simulink library "powerlib2"  (Simulink 6.0)
settings: Solver=ode45  SolverMode=SingleTasking  StartTime=0.0  StopTime=10.0  RelTol=1e-3
undefined symbols (not defined in the file or in its folder): com, ctrl1, Da, DiscIntNeverNeededParam, dtha, etat, FA, gcbh, Ha, Ka, Lm, Ls, powericonV2, q0, Rm, Rs, sel, st_a, st_b, st_c, sta, stb, stc, T1, T2, T3, T4
libraries: powerlib2 x55, simulink_extras x5, powerlib_extras x4, powerlib_modelsV2 x4, simulink x1
(part 5 of 6)

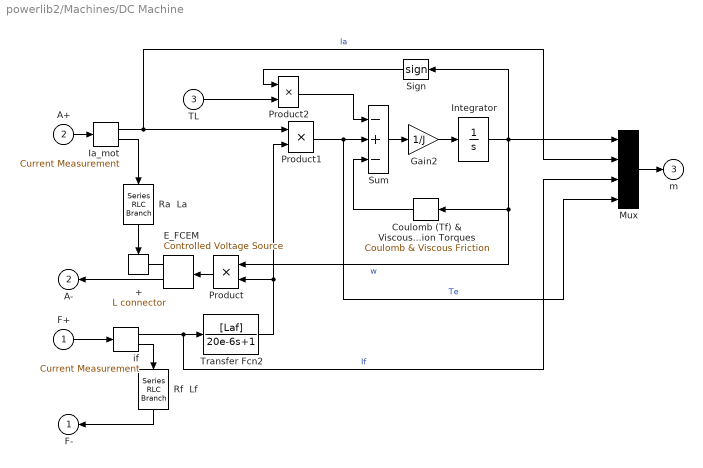
== system powerlib2/Machines/DC Machine ==
  F+ : Inport  Port=1  LatchInput=off
  A+ : Inport  Port=2  LatchInput=off
  TL : Inport  Port=3  LatchInput=off
  + : powerlib2/Connectors/L connector  Tag=PoWeRsYsTeMbLoCk  Orientation=down
  Coulomb (Tf) & Viscous ( Bm*w)  Friction Torques : simulink/Discontinuities/Coulomb & Viscous Friction  Orientation=left  offset=Tf  gain=Bm
  E_FCEM : powerlib2/Electrical Sources/Controlled Voltage Source  Tag=PoWeRsYsTeMbLoCk  Orientation=left  initsrc=on  srctyp=AC  iv=0  iph=0  ifreq=0  mesure=None  PSBOutputType=11
  Gain2 : Gain  Gain=1/J  SaturateOnIntegerOverflow=on
  Ia_mot : powerlib2/Measurements/Current Measurement  Tag=PoWeRsYsTeMmEaSuReMeNtFiRsT  PhasorSimulation=off  OutputType=Magnitude  PSBOutputType=01  PSBequivalent=0
  Integrator : Integrator  InitialCondition=w0
  Mux : Mux
  Product : Product  Orientation=left  SaturateOnIntegerOverflow=on  InputSameDT=on
  Product1 : Product  SaturateOnIntegerOverflow=on  InputSameDT=on
  Product2 : Product  SaturateOnIntegerOverflow=on  InputSameDT=on
  Ra  La : powerlib2/Elements/Series RLC Branch  Tag=PoWeRsYsTeMbLoCk  Orientation=down  a=Ra  b=La  c=inf  mesure=None  PSBOutputType=1
  Rf  Lf : powerlib2/Elements/Series RLC Branch  Tag=PoWeRsYsTeMbLoCk  Orientation=down  a=Rf  b=Lf  c=inf  mesure=None  PSBOutputType=1
  Sign : Signum  Orientation=left
  Sum : Sum  Inputs=-+-  SaturateOnIntegerOverflow=on  InputSameDT=on
  Transfer Fcn2 : TransferFcn  Numerator=[Laf]  Denominator=[20e-6 1]
  if : powerlib2/Measurements/Current Measurement  Tag=PoWeRsYsTeMmEaSuReMeNt  PhasorSimulation=off  OutputType=Magnitude  PSBOutputType=01  PSBequivalent=0
  F- : Outport  Orientation=left  InitialOutput=0
  A- : Outport  Orientation=left  Port=2  InitialOutput=0
  m : Outport  Port=3  InitialOutput=0
  wires:
  A+/1 -> Ia_mot/1
  Ia_mot/2 -> Ra  La/1
  Ra  La/1 -> +/1
  F+/1 -> if/1
  if/2 -> Rf  Lf/1
  E_FCEM/1 -> +/Enable
  E_FCEM/2 -> A-/1
  Rf  Lf/1 -> F-/1
  Ia_mot/1 -> Product1/1, Mux/2  "Ia"
  if/1 -> Transfer Fcn2/1, Mux/3  "If"
  Product2/1 -> Sum/1
  TL/1 -> Product2/2
  Sign/1 -> Product2/1
  Sum/1 -> Gain2/1
  Gain2/1 -> Integrator/1
  Integrator/1 -> Coulomb (Tf) & Viscous ( Bm*w)  Friction Torques/1, Product/1, Mux/1, Sign/1  "w"
  Product/1 -> E_FCEM/1
  Product1/1 -> Sum/2, Mux/4  "Te"
  Mux/1 -> m/1
  Transfer Fcn2/1 -> Product1/2, Product/2
  Coulomb (Tf) & Viscous ( Bm*w)  Friction Torques/1 -> Sum/3

== system powerlib2/Machines/Excitation System ==
  vref : Inport  Port=1  LatchInput=off
  vd : Inport  Port=2  LatchInput=off
  vq : Inport  Port=3  LatchInput=off
  vstab : Inport  Port=4  LatchInput=off
  Source : powerlib_modelsV2/Continuous/Excitation_System  tr=tr  reg=reg  exc=exc  tgr=tgr  damp=damp  sat=sat  lim=lim  v0=v0
  Vf : Outport  InitialOutput=0
  wires:
  Source/1 -> Vf/1
  vref/1 -> Source/1
  vd/1 -> Source/2
  vq/1 -> Source/3
  vstab/1 -> Source/4

== system powerlib2/Machines/Generic Power System Stabilizer ==
  In : Inport  Port=1  LatchInput=off
  Source : powerlib_modelsV2/Continuous/PSS  Tsensor=Tsensor  K=K  Twashout=Twashout  Tleadlag1=Tleadlag1  Tleadlag2=Tleadlag2  VSlimits=VSlimits  Vinit=Vinit  Plot_On=off  MagdB_On=on  FreqRange=logspace(-2,2,500)
  Vstab : Outport  InitialOutput=0
  wires:
  Source/1 -> Vstab/1
  In/1 -> Source/1

== system powerlib2/Machines/HTG ==
  wref : Inport  Port=1  LatchInput=off
  Pref : Inport  Port=2  LatchInput=off
  we : Inport  Port=3  LatchInput=off
  Pe0 : Inport  Port=4  LatchInput=off
  dw : Inport  Port=5  LatchInput=off
  Source : powerlib_modelsV2/Continuous/HTG  sm=sm  gate=gate  reg=reg  hyd=hyd  dref=dref  po=po
  Pm : Outport  InitialOutput=0
  gate : Outport  Port=2  InitialOutput=0
  wires:
  wref/1 -> Source/1
  Pref/1 -> Source/2
  we/1 -> Source/3
  Pe0/1 -> Source/4
  dw/1 -> Source/5
  Source/2 -> gate/1
  Source/1 -> Pm/1

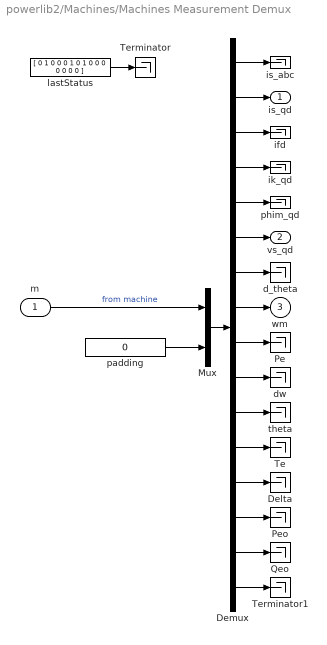
== system powerlib2/Machines/Machines Measurement Demux ==
  m : Inport  Port=1  LatchInput=off
  Delta : Terminator
      settings: Tag=port13
  Demux : Demux  Outputs="[3 2 1 3 2 2 1 1 1 1 1 1 1 1 1,  1]"
  Mux : Mux  Inputs=2
  Pe : Terminator
      settings: Tag=port9
  Peo : Terminator
      settings: Tag=port14
  Qeo : Terminator
      settings: Tag=port15
  Te : Terminator
      settings: Tag=port12
  Terminator : Terminator
  Terminator1 : Terminator
  d_theta : Terminator
      settings: Tag=port7
  dw : Terminator
      settings: Tag=port10
  ifd : Terminator
      settings: Tag=port3
  ik_qd : Terminator
      settings: Tag=port4
  is_abc : Terminator
      settings: Tag=port1
  lastStatus : Constant  Value="[ 0  1  0  0  0  1  0  1  0  0  0  0  0  0  0 ]"
  padding : Constant  Value=0
  phim_qd : Terminator
      settings: Tag=port5
  theta : Terminator
      settings: Tag=port11
  is_qd : Outport  Tag=port2
  vs_qd : Outport  Tag=port6  Port=2
  wm : Outport  Tag=port8  Port=3
  wires:
  padding/1 -> Mux/2
  Demux/1 -> is_abc/1
  Demux/2 -> is_qd/1
  Demux/3 -> ifd/1
  Demux/4 -> ik_qd/1
  Demux/5 -> phim_qd/1
  Demux/6 -> vs_qd/1
  Demux/7 -> d_theta/1
  Demux/8 -> wm/1
  Demux/9 -> Pe/1
  Demux/10 -> dw/1
  Demux/11 -> theta/1
  Mux/1 -> Demux/1
  lastStatus/1 -> Terminator/1
  m/1 -> Mux/1  "from machine"
  Demux/16 -> Terminator1/1
  Demux/15 -> Qeo/1
  Demux/14 -> Peo/1
  Demux/13 -> Delta/1
  Demux/12 -> Te/1

== system powerlib2/Machines/Multi-Band Power System Stabilizer ==
  dw : Inport  Port=1  LatchInput=off
  Source : powerlib_modelsV2/Continuous/MBPSS  OperationMode=Simplified settings  Kg=Kg  GL=GL  GI=GI  GH=GH  GLd=GLd  TcLF=TcLF  GId=GId  TcIF=TcIF  GHd=GHd  TcHF=TcHF  LIM=LIM  Plot_On=off  MagdB_On=off  FreqRange=logspace(-2,2,500)
  Vstab : Outport  InitialOutput=0
  wires:
  dw/1 -> Source/1
  Source/1 -> Vstab/1

== system powerlib2/Machines/Permanent Magnet Synchronous Machine ==
  A : Inport  Port=1  LatchInput=off
  B : Inport  Port=2  LatchInput=off
  C : Inport  Port=3  LatchInput=off
  Tm : Inport  Port=4  LatchInput=off
  Terminator : Terminator
  Terminator1 : Terminator
  Terminator2 : Terminator
  m : Outport  InitialOutput=0
  tag scope: tp200482=global
  wires:
  C/1 -> Terminator2/1
  B/1 -> Terminator1/1
  A/1 -> Terminator/1
  Tm/1 -> [tp200482]
  [tp200488] -> m/1

== system powerlib2/Machines/STG ==
  wref : Inport  Port=1  LatchInput=off
  Pref : Inport  Port=2  LatchInput=off
  wm : Inport  Port=3  LatchInput=off
  d_theta : Inport  Port=4  LatchInput=off
  4 mass shaft : Subsystem  TreatAsAtomicUnit=on
  Constant2 : Constant  Orientation=up  Value=gentype==2
  Constant3 : Constant  Orientation=up  Value=gentype~=2
  Pboil : Constant  Orientation=left  Value=1.0
  Product : Product  SaturateOnIntegerOverflow=on  InputSameDT=on
  Sum : Sum  Inputs=+  SaturateOnIntegerOverflow=on  InputSameDT=on
  Switch1 : Switch  Threshold=0.5  InputSameDT=on
  speed regulator : Subsystem  mask(Speed regulator for thermal turbine){Rp=reg1(2), Kp=reg1(1), Dz=reg1(3), Tsr=reg2(1), Tsm=reg2(2), lim=reg3, g0=q0}
      mask prompts: Rp "Permanent droop Rp:"; Kp "Regulator gain Kp:"; Dz "Regulator dead zone limit Dz (p.u.):"; Tsr "Speed relay time constant Tsr (s):"; Tsm "Servo motor time constant Tsv:"; lim "Gate opening limits [ vgmin,vgmax (p.u./s)  gmin,gmax (p.u.)]:"; g0 "Initial gate opening g0 (p.u.):"
      mask init:
      | vgmin=lim(1); vgmax=lim(2); gmin=lim(3); gmax=lim(4);
  steam turbine : Subsystem  mask(Thermal turbine){Fa=FA, Ta=turb1, f0=q0}
      mask prompts: Fa "Generator 1 torque fractions [ F1  F2  F3  F4 ]:"; Ta "Time constants [ T1  T2  T3  T4 ] (s):"; f0 "Initial flows f0:"
      mask init:
      | F2=Fa(1); F3=Fa(2); F4=Fa(3); F5=Fa(4);
      | if Ta(1)==0, T1=1; else T1=Ta(1); end; if Ta(2)==0, T2=1; else T2=Ta(2); end
      | if Ta(3)==0, T3=1; else T3=Ta(3); end; if Ta(4)==0, T4=1; else T4=Ta(4); end
  dw_5-2 : Outport
  Tr5-2 : Outport  Port=2
  gate : Outport  Port=3
  Pm : Outport  Port=4
  wires:
  wm/1 -> Product/2, speed regulator/4(w)
  Pref/1 -> speed regulator/2(Pref)
  wref/1 -> speed regulator/3(wref)
  Pboil/1 -> steam turbine/2(Pboil)
  Product/1 -> Pm/1
  4 mass shaft/2(Tr2-5) -> Tr5-2/1
  Switch1/1 -> Product/1
  4 mass shaft/1(Tm_g) -> Switch1/3
  Sum/1 -> Switch1/1
  Constant3/1 -> Switch1/2
  d_theta/1 -> 4 mass shaft/2(d_theta)
  steam turbine/1(flowHp) -> speed regulator/1(flowHP)
  steam turbine/2(T5-2) -> 4 mass shaft/1(T5-2), Sum/1
  4 mass shaft/3(dw_5-2) -> dw_5-2/1
  speed regulator/1(gate opening) -> steam turbine/1(gate), gate/1
  Constant2/1 -> 4 mass shaft/Enable

== system powerlib2/Machines/Simplified Synchronous  Machine  pu Units ==
  Pm : Inport  Port=1  LatchInput=off
  E : Inport  Port=2  LatchInput=off
  Constant{,1..3} (4 alike) : Constant
  N : Terminator
  A : Outport  InitialOutput=0
  B : Outport  Port=2  InitialOutput=0
  C : Outport  Port=3  InitialOutput=0
  m_pu : Outport  Port=4  InitialOutput=0
  tag scope: tp200493=global, tp200499=global
  wires:
  [tp200504] -> m_pu/1
  Constant3/1 -> N/1
  Pm/1 -> [tp200493]
  E/1 -> [tp200499]
  Constant2/1 -> C/1
  Constant1/1 -> B/1
  Constant/1 -> A/1

== system powerlib2/Machines/Simplified Synchronous  Machine SI Units ==
  Pm : Inport  Port=1  LatchInput=off
  E : Inport  Port=2  LatchInput=off
  Constant{,1..3} (4 alike) : Constant
  N : Terminator
  A : Outport  InitialOutput=0
  B : Outport  Port=2  InitialOutput=0
  C : Outport  Port=3  InitialOutput=0
  m_SI : Outport  Port=4  InitialOutput=0
  tag scope: tp200509=global, tp200515=global
  wires:
  Constant3/1 -> N/1
  Constant2/1 -> C/1
  [tp200521] -> m_SI/1
  Constant/1 -> A/1
  Constant1/1 -> B/1
  Pm/1 -> [tp200509]
  E/1 -> [tp200515]

== system powerlib2/Machines/Synchronous Machine SI Fundamental ==
  Pm : Inport  Port=1  LatchInput=off
  Vf : Inport  Port=2  LatchInput=off
  Constant : Constant
  Constant1 : Constant
  Constant2 : Constant
  A : Outport  InitialOutput=0
  B : Outport  Port=2  InitialOutput=0
  C : Outport  Port=3  InitialOutput=0
  m_SI : Outport  Port=4  InitialOutput=0
  tag scope: tp200526=global, tp200532=global
  wires:
  Vf/1 -> [tp200532]
  Pm/1 -> [tp200526]
  [tp200537] -> m_SI/1
  Constant/1 -> A/1
  Constant1/1 -> B/1
  Constant2/1 -> C/1

== system powerlib2/Machines/Synchronous Machine pu Fundamental ==
  Pm : Inport  Port=1  LatchInput=off
  Vf : Inport  Port=2  LatchInput=off
  Constant : Constant
  Constant1 : Constant
  Constant2 : Constant
  A : Outport  InitialOutput=0
  B : Outport  Port=2  InitialOutput=0
  C : Outport  Port=3  InitialOutput=0
  m_pu : Outport  Port=4  InitialOutput=0
  tag scope: tp200543=global, tp200548=global
  wires:
  [tp200554] -> m_pu/1
  Pm/1 -> [tp200543]
  Vf/1 -> [tp200548]
  Constant/1 -> A/1
  Constant1/1 -> B/1
  Constant2/1 -> C/1

== system powerlib2/Machines/Synchronous Machine pu Standard ==
  Pm : Inport  Port=1  LatchInput=off
  Vf : Inport  Port=2  LatchInput=off
  Constant : Constant
  Constant1 : Constant
  Constant2 : Constant
  A : Outport  InitialOutput=0
  B : Outport  Port=2  InitialOutput=0
  C : Outport  Port=3  InitialOutput=0
  m_pu : Outport  Port=4  InitialOutput=0
  tag scope: tp200559=global, tp200565=global
  wires:
  Vf/1 -> [tp200565]
  Pm/1 -> [tp200559]
  [tp200570] -> m_pu/1
  Constant/1 -> A/1
  Constant1/1 -> B/1
  Constant2/1 -> C/1

== system powerlib2/Measurements/Current Measurement ==
  + : Inport  Port=1  LatchInput=off
  Constant : Constant  Orientation=left
  Mux : Mux  Inputs=2
  Phasor Measurements : powerlib2/Measurements/Voltage Measurement/Phasor Measurements  TreatAsAtomicUnit=on  SimViewingDevice=off  DataTypeOverride=UseLocalSettings  MinMaxOverflowLogging=UseLocalSettings
      settings: Permissions=ReadWrite  RTWFcnNameOpts=Auto  RTWFileNameOpts=Auto
  Selector : Selector  Elements=SelectionMode  InputPortWidth=length(OutputSelection)+1
  Simulation method : Constant  Orientation=down  Value=PhasorSimulation
  Terminator : Terminator
  i : Outport  InitialOutput=0
  - : Outport  Orientation=left  Port=2  InitialOutput=0
  wires:
  +/1 -> Terminator/1
  Constant/1 -> -/1
  Simulation method/1 -> Phasor Measurements/Enable
  Mux/1 -> Selector/1
  Phasor Measurements/1 -> Mux/1
  [tp200576] -> Phasor Measurements/1, Mux/2
  Selector/1 -> i/1

== system powerlib2/Measurements/Extra Library  ==

== system powerlib2/Measurements/Extra Library 1 ==

== system powerlib2/Measurements/Impedance Measurement ==
  note: Use this block
      | with the powergui
      | interface
  1 : Inport  Port=1  LatchInput=off
  2 : Inport  Port=2  LatchInput=off
  Terminator : Terminator
  Terminator1 : Terminator
  wires:
  2/1 -> Terminator1/1
  1/1 -> Terminator/1

== system powerlib2/Measurements/Multimeter ==
  Gain2 : Gain  Gain=Gain  SaturateOnIntegerOverflow=on
  Mode : Constant  Value=Display
  Mux : Mux  Inputs=2
  Phasor Measurements : Subsystem  TreatAsAtomicUnit=on
  Selector : Selector  Elements=SelectionMode  InputPortWidth=length(OutputSelection)+length(sel)
  Simulation method : Constant  Orientation=down  Value=PhasorSimulation
  StoreData : Subsystem  Orientation=down  LoadFcn=if strcmp(bdroot,'powerlib')|strcmp(bdroot,'powerlib11')|strcmp(bdroot,'powerlib2');return;else;set_param([gcb,'/To Workspace'],'VariableName',strrep(tempname,tempdir,''));end  TreatAsAtomicUnit=on  mask{RowMax=inf}
      mask prompts: RowMax "Maximum Number of rows"
      settings: CopyFcn=if strcmp(bdroot,'powerlib')|strcmp(bdroot,'powerlib11')|strcmp(bdroot,'powerlib2');return;else;set_param([gcb,'/To Workspace'],'VariableName',strrep(tempname,tempdir,''));end
  selection : Selector  Elements=sel  InputPortWidth=L
  Out1 : Outport
  wires:
  Mode/1 -> StoreData/Enable
  selection/1 -> Gain2/1
  [gotomultimeterPSB] -> selection/1
  Gain2/1 -> Phasor Measurements/1(In1), Mux/2
  Simulation method/1 -> Phasor Measurements/Enable
  Phasor Measurements/1(Out1) -> Mux/1
  Mux/1 -> Selector/1
  Selector/1 -> Out1/1, StoreData/1(In1)

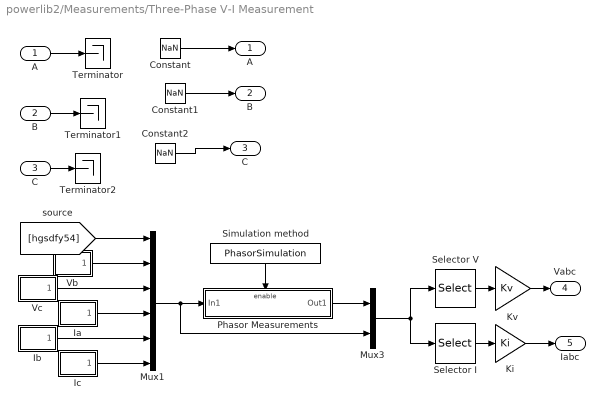
== system powerlib2/Measurements/Three-Phase V-I Measurement ==
  A : Inport  Port=1  LatchInput=off
  B : Inport  Port=2  LatchInput=off
  C : Inport  Port=3  LatchInput=off
  Constant : Constant  Value=NaN
  Constant1 : Constant  Value=NaN
  Constant2 : Constant  Value=NaN
  Ia : Subsystem
  Ib : Subsystem
  Ic : Subsystem
  Ki : Gain  Gain=Ki  SaturateOnIntegerOverflow=on
  Kv : Gain  Gain=Kv  SaturateOnIntegerOverflow=on
  Mux1 : Mux  Inputs=6
  Mux3 : Mux  Inputs=2
  Phasor Measurements : Subsystem  TreatAsAtomicUnit=on
  Selector I : Selector  Elements=SelectionModeI  InputPortWidth=length(OutputSelection)+6
  Selector V : Selector  Elements=SelectionModeV  InputPortWidth=length(OutputSelection)+6
  Simulation method : Constant  Orientation=down  Value=PhasorSimulation
  Terminator : Terminator
  Terminator1 : Terminator
  Terminator2 : Terminator
  Vb : Subsystem
  Vc : Subsystem
  "A " : Outport
  "B " : Outport  Port=2
  "C " : Outport  Port=3
  Vabc : Outport  Port=4
  Iabc : Outport  Port=5
  wires:
  A/1 -> Terminator/1
  B/1 -> Terminator1/1
  C/1 -> Terminator2/1
  Constant/1 -> "A "/1
  Constant1/1 -> "B "/1
  Constant2/1 -> "C "/1
  Kv/1 -> Vabc/1
  Ki/1 -> Iabc/1
  Selector V/1 -> Kv/1
  Selector I/1 -> Ki/1
  Mux3/1 -> Selector I/1, Selector V/1
  Phasor Measurements/1(Out1) -> Mux3/1
  Simulation method/1 -> Phasor Measurements/Enable
  Mux1/1 -> Mux3/2, Phasor Measurements/1(In1)
  [hgsdfy54] -> Mux1/1
  Vb/1(Out1) -> Mux1/2
  Vc/1(Out1) -> Mux1/3
  Ia/1(Out1) -> Mux1/4
  Ib/1(Out1) -> Mux1/5
  Ic/1(Out1) -> Mux1/6

== system powerlib2/Measurements/Voltage Measurement ==
  + : Inport  Port=1  LatchInput=off
  - : Inport  Port=2  LatchInput=off
  Mux : Mux  Inputs=2
  Phasor Measurements : Subsystem  TreatAsAtomicUnit=on
  Selector : Selector  Elements=SelectionMode  InputPortWidth=length(OutputSelection)+1
  Simulation method : Constant  Orientation=down  Value=PhasorSimulation
  Terminator : Terminator
  Terminator1 : Terminator
  v : Outport  InitialOutput=0
  wires:
  Simulation method/1 -> Phasor Measurements/Enable
  Mux/1 -> Selector/1
  Phasor Measurements/1(options) -> Mux/1
  Selector/1 -> v/1
  -/1 -> Terminator1/1
  +/1 -> Terminator/1
  [tp200597] -> Mux/2, Phasor Measurements/1(measure)

== system powerlib2/Power Electronics/  Extra Library  ==

== system powerlib2/Power Electronics/  Extra Library 1 ==

== system powerlib2/Power Electronics/Detailed Thyristor ==
  a : Inport  Port=1  LatchInput=off
  g : Inport  Port=2  LatchInput=off
  Constant : Constant
  Terminator : Terminator
  k : Outport  InitialOutput=0
  m : Outport  Port=2  InitialOutput=0
  tag scope: tp200603=global
  wires:
  a/1 -> Terminator/1
  Constant/1 -> k/1
  g/1 -> [tp200603]
  [tp200608] -> m/1

== system powerlib2/Power Electronics/Diode ==
  a : Inport  Port=1  LatchInput=off
  Constant : Constant
  Terminator : Terminator
  k : Outport  InitialOutput=0
  m : Outport  Port=2  InitialOutput=0
  wires:
  a/1 -> Terminator/1
  Constant/1 -> k/1
  [tp200614] -> m/1

== system powerlib2/Power Electronics/Gto ==
  a : Inport  Port=1  LatchInput=off
  g : Inport  Port=2  LatchInput=off
  Constant : Constant
  Terminator : Terminator
  k : Outport  InitialOutput=0
  m : Outport  Port=2  InitialOutput=0
  tag scope: tp200619=global
  wires:
  a/1 -> Terminator/1
  Constant/1 -> k/1
  g/1 -> [tp200619]
  [tp200625] -> m/1

== system powerlib2/Power Electronics/IGBT ==
  C : Inport  Port=1  LatchInput=off
  g : Inport  Port=2  LatchInput=off
  Constant : Constant
  Terminator : Terminator
  E : Outport  InitialOutput=0
  m : Outport  Port=2  InitialOutput=0
  tag scope: tp200630=global
  wires:
  [tp200636] -> m/1
  g/1 -> [tp200630]
  Constant/1 -> E/1
  C/1 -> Terminator/1

== system powerlib2/Power Electronics/Ideal Switch ==
  1 : Inport  Port=1  LatchInput=off
  g : Inport  Port=2  LatchInput=off
  Constant : Constant
  Terminator : Terminator
  2 : Outport  InitialOutput=0
  m : Outport  Port=2  InitialOutput=0
  tag scope: tp200641=global
  wires:
  [tp200647] -> m/1
  g/1 -> [tp200641]
  Constant/1 -> 2/1
  1/1 -> Terminator/1

== system powerlib2/Power Electronics/Mosfet ==
  d : Inport  Port=1  LatchInput=off
  g : Inport  Port=2  LatchInput=off
  Constant : Constant
  Terminator : Terminator
  s : Outport  InitialOutput=0
  m : Outport  Port=2  InitialOutput=0
  tag scope: tp200652=global
  wires:
  [tp200658] -> m/1
  g/1 -> [tp200652]
  Constant/1 -> s/1
  d/1 -> Terminator/1

== system powerlib2/Power Electronics/Three-Level Bridge ==
  A : Inport  Port=1  LatchInput=off
  B : Inport  Port=2  LatchInput=off
  C : Inport  Port=3  LatchInput=off
  pulses : Inport  Port=4  PortDimensions=4*arms  LatchInput=off
  Logical Operator : Logic  OutDataTypeMode=Specify via dialog  LogicDataType=float('double')
  c1 : Constant
  c2 : Constant
  c3 : Constant
  s1 : Selector  Elements=selection1  InputPortWidth=4*arms
  s2 : Selector  Elements=selection2  InputPortWidth=4*arms
  t1 : Terminator
  t2 : Terminator
  t3 : Terminator
  + : Outport  InitialOutput=0
  N : Outport  Port=2  InitialOutput=0
  - : Outport  Port=3  InitialOutput=0
  tag scope: tp420660=global
  wires:
  pulses/1 -> s2/1, s1/1
  Logical Operator/1 -> [tp420660]
  s2/1 -> Logical Operator/2
  s1/1 -> Logical Operator/1
  c3/1 -> -/1
  c2/1 -> N/1
  c1/1 -> +/1
  C/1 -> t3/1
  B/1 -> t2/1
  A/1 -> t1/1

== system powerlib2/Power Electronics/Thyristor ==
  a : Inport  Port=1  LatchInput=off
  g : Inport  Port=2  LatchInput=off
  Constant : Constant
  Terminator : Terminator
  k : Outport  InitialOutput=0
  m : Outport  Port=2  InitialOutput=0
  tag scope: tp200663=global
  wires:
  a/1 -> Terminator/1
  Constant/1 -> k/1
  g/1 -> [tp200663]
  [tp200669] -> m/1

== system powerlib2/Power Electronics/Universal Bridge ==
  A : Inport  Port=1  LatchInput=off
  B : Inport  Port=2  LatchInput=off
  C : Inport  Port=3  LatchInput=off
  pulses : Inport  Port=4  PortDimensions=2*arms  LatchInput=off
  c1 : Constant
  c2 : Constant
  c3 : Constant
  o3 : Terminator
  t1 : Terminator
  t2 : Terminator
  t3 : Terminator
  + : Outport  InitialOutput=0
  - : Outport  Port=2  InitialOutput=0
  tag scope: tp200674=global
  wires:
  c3/1 -> o3/1
  c2/1 -> -/1
  c1/1 -> +/1
  C/1 -> t3/1
  B/1 -> t2/1
  A/1 -> t1/1
  pulses/1 -> [tp200674]

== system powerlib2/powergui/Subsystem ==

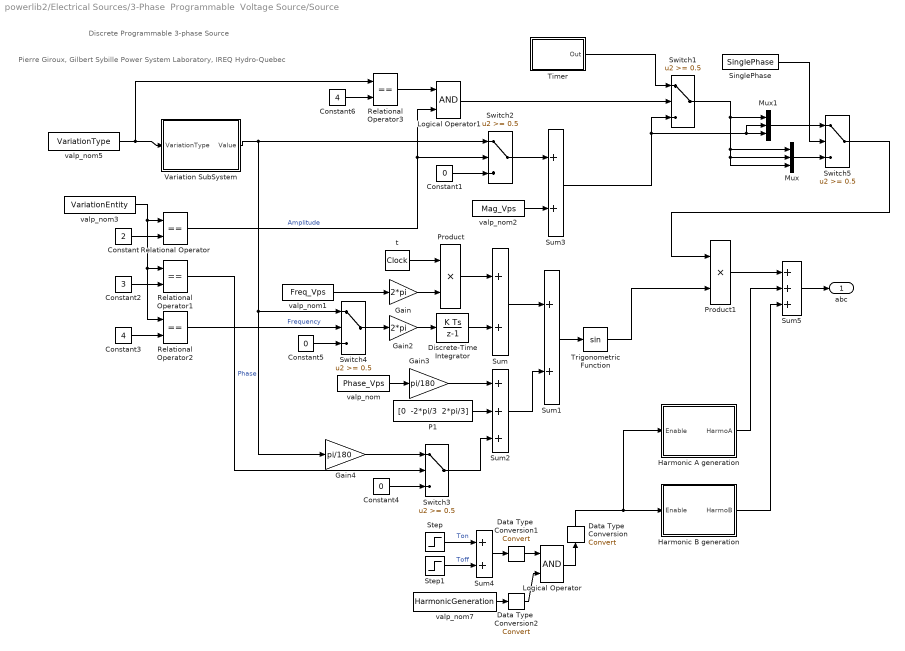
== system powerlib2/Electrical Sources/3-Phase  Programmable  Voltage Source/Source ==
  note: Discrete Programmable 3-phase Source
  note: Pierre Giroux, Gilbert Sybille
      | Power System Laboratory, IREQ
      | Hydro-Quebec
  Constant : Constant  Value=2
  Constant1 : Constant  Value=0
  Constant2 : Constant  Value=3
  Constant3 : Constant  Value=4
  Constant4 : Constant  Value=0
  Constant5 : Constant  Value=0
  Constant6 : Constant  Value=4
  Data Type  Conversion : DataTypeConversion  Orientation=up  OutDataTypeMode=double  SaturateOnIntegerOverflow=on  RndMeth=Zero
  Data Type  Conversion1 : DataTypeConversion  OutDataTypeMode=boolean  SaturateOnIntegerOverflow=on  RndMeth=Zero
  Data Type  Conversion2 : DataTypeConversion  OutDataTypeMode=boolean  SaturateOnIntegerOverflow=on  RndMeth=Zero
  Discrete-Time Integrator : DiscreteIntegrator  SampleTime=Ts  ICPrevOutput=DiscIntNeverNeededParam  ICPrevScaledInput=DiscIntNeverNeededParam
  Gain : Gain  Gain=2*pi  SaturateOnIntegerOverflow=on
  Gain2 : Gain  Gain=2*pi  SaturateOnIntegerOverflow=on
  Gain3 : Gain  Gain=pi/180  SaturateOnIntegerOverflow=on
  Gain4 : Gain  Gain=pi/180  SaturateOnIntegerOverflow=on
  Harmonic A generation : Subsystem  mask(Harmonic generation){Freq_Vps=Freq_Vps, n_Harmo=n_HarmoA, Mag_Harmo=Mag_HarmoA, Phase_Harmo=Phase_HarmoA, Seq_Harmo=Seq_HarmoA, Ts=Ts}
      mask prompts: Ts "Sample time:"
  Harmonic B generation : Subsystem  mask(Harmonic generation){Freq_Vps=Freq_Vps, n_Harmo=n_HarmoB, Mag_Harmo=Mag_HarmoB, Phase_Harmo=Phase_HarmoB, Seq_Harmo=Seq_HarmoB, Ts=Ts}
      mask prompts: Ts "Sample time:"
  Logical Operator : Logic
  Logical Operator1 : Logic
  Mux : Mux  Inputs=3
  Mux1 : Mux  Inputs=3
  P1 : Constant  Value="[0  -2*pi/3  2*pi/3]"
  Product : Product  SaturateOnIntegerOverflow=on  InputSameDT=on
  Product1 : Product  SaturateOnIntegerOverflow=on  InputSameDT=on
  Relational Operator{,1..3} (4 alike) : RelationalOperator  Operator===  InputSameDT=on
  SinglePhase : Constant  Value=SinglePhase
  Step : Step  Time=Ton_Harmo  SampleTime=Ts
  Step1 : Step  Time=Toff_Harmo  After=-1  SampleTime=Ts
  Sum{,1,3..4} (4 alike) : Sum  SaturateOnIntegerOverflow=on  InputSameDT=on
  Sum2 : Sum  Inputs=+++  SaturateOnIntegerOverflow=on  InputSameDT=on
  Sum5 : Sum  Inputs=+++  SaturateOnIntegerOverflow=on  InputSameDT=on
  Switch{1..5} (5 alike) : Switch  Threshold=0.5  InputSameDT=on
  Timer : Subsystem  mask(Timer){t=Xtime, e=Yampli}
      mask prompts: t "Time (s):"; e "Amplitude:"
      mask help:
      | Generates a signal changing  at specified times.
      |
      | Value of the signal at time zero must  be specified.
      mask init:
      | tt=t;sv=e;
      | tv=[-1,tt(1),reshape(repmat(reshape(tt(2:end),1,length(tt)-1),2,1),1,2*length(tt)-2),tt(end)+1];
      | %sv=(sv(:)'~=0);
      | opv=[sv(1),reshape(repmat(sv(1:end-1),2,1),1,2*length(sv)-2),sv(end),sv(end)];
      mask Display: plot( tv(2:end-1), opv(2:end-1) )
  Trigonometric Function : Trigonometry
  Variation SubSystem : Subsystem  mask(Variation Subsystem){VariationStep=VariationStep, VariationRate=VariationRate, VariationFreq=VariationFreq, VariationMag=VariationMag, Ton_Variation=Ton_Variation, Toff_Variation=Toff_Variation, Ts=Ts}
      mask prompts: Ts "Sample time:"
  t : DigitalClock  SampleTime=Ts
  valp_nom : Constant  Value=Phase_Vps
  valp_nom1 : Constant  Value=Freq_Vps
  valp_nom2 : Constant  Value=Mag_Vps
  valp_nom3 : Constant  Value=VariationEntity
  valp_nom5 : Constant  Value=VariationType
  valp_nom7 : Constant  Value=HarmonicGeneration
  abc : Outport  InitialOutput=0
  wires:
  Data Type  Conversion2/1 -> Logical Operator/2
  valp_nom7/1 -> Data Type  Conversion2/1
  Data Type  Conversion1/1 -> Logical Operator/1
  Sum4/1 -> Data Type  Conversion1/1
  Data Type  Conversion/1 -> Harmonic B generation/1(Enable), Harmonic A generation/1(Enable)
  Logical Operator/1 -> Data Type  Conversion/1
  Product/1 -> Sum/1
  Gain/1 -> Product/2
  t/1 -> Product/1
  Sum/1 -> Sum1/1
  Sum1/1 -> Trigonometric Function/1
  Gain2/1 -> Discrete-Time Integrator/1
  Discrete-Time Integrator/1 -> Sum/2
  P1/1 -> Sum2/2
  Trigonometric Function/1 -> Product1/2
  Gain3/1 -> Sum2/1
  valp_nom/1 -> Gain3/1
  valp_nom1/1 -> Gain/1
  Product1/1 -> Sum5/1
  Switch2/1 -> Sum3/1
  Constant1/1 -> Switch2/3
  Sum2/1 -> Sum1/2
  valp_nom2/1 -> Sum3/2
  Relational Operator/1 -> Switch2/2, Logical Operator1/2  "Amplitude"
  valp_nom5/1 -> Variation SubSystem/1(VariationType), Relational Operator3/1
  Switch3/1 -> Sum2/3
  Constant4/1 -> Switch3/3
  Relational Operator1/1 -> Switch3/2  "Phase"
  Variation SubSystem/1(Value) -> Switch2/1, Switch4/1, Gain4/1
  Switch4/1 -> Gain2/1
  Relational Operator2/1 -> Switch4/2  "Frequency"
  Constant/1 -> Relational Operator/2
  valp_nom3/1 -> Relational Operator/1, Relational Operator2/1, Relational Operator1/1
  Constant2/1 -> Relational Operator1/2
  Constant3/1 -> Relational Operator2/2
  Constant5/1 -> Switch4/3
  Harmonic A generation/1(HarmoA) -> Sum5/2
  Sum5/1 -> abc/1
  Step/1 -> Sum4/1  "Ton"
  Step1/1 -> Sum4/2  "Toff"
  Harmonic B generation/1(HarmoB) -> Sum5/3
  Gain4/1 -> Switch3/1
  Constant6/1 -> Relational Operator3/2
  Sum3/1 -> Switch1/3, Mux1/3, Mux1/2
  Timer/1(Out) -> Switch1/1
  Mux1/1 -> Switch5/1
  SinglePhase/1 -> Switch5/2
  Mux/1 -> Switch5/3
  Switch1/1 -> Mux/1, Mux/2, Mux/3, Mux1/1
  Switch5/1 -> Product1/1
  Relational Operator3/1 -> Logical Operator1/1
  Logical Operator1/1 -> Switch1/2

== system powerlib2/Machines/STG/4 mass shaft ==
  T5-2 : Inport  Port=1  LatchInput=off
  d_theta : Inport  Port=2  LatchInput=off
  Enable : EnablePort
  1 mass : Subsystem  TreatAsAtomicUnit=on
  2 masses : Subsystem  TreatAsAtomicUnit=on
  3 masses : Subsystem  TreatAsAtomicUnit=on
  4 masses : Subsystem  TreatAsAtomicUnit=on
  Multiport Switch1 : MultiPortSwitch  InputSameDT=on
  Multiport Switch2 : MultiPortSwitch  InputSameDT=on
  Multiport Switch3 : MultiPortSwitch  InputSameDT=on
  ctrl2 : Constant  Orientation=down  Value=ctrl1==4
  ctrl3 : Constant  Orientation=down  Value=ctrl1==3
  ctrl4 : Constant  Orientation=left  Value=ctrl1
  ctrl6 : Constant  Orientation=down  Value=ctrl1==2
  ctrl7 : Constant  Orientation=down  Value=ctrl1==1
  Tm_g : Outport  OutputWhenDisabled=reset  InitialOutput=0
  Tr2-5 : Outport  Port=2  OutputWhenDisabled=reset  InitialOutput=[0 0 0 0]
  dw_5-2 : Outport  Port=3  OutputWhenDisabled=reset  InitialOutput=[0 0 0 0]
  wires:
  1 mass/1(Ts_5-2) -> Multiport Switch1/2
  2 masses/1(Ts_5-2) -> Multiport Switch1/3
  3 masses/1(Ts_5-2) -> Multiport Switch1/4
  4 masses/1(Ts_5-2) -> Multiport Switch1/5
  T5-2/1 -> 1 mass/1(Tt_1-4), 2 masses/1(Tt_1-4), 3 masses/1(Tt_1-4), 4 masses/1(Tt_1-4)
  d_theta/1 -> 1 mass/2(dth_gen), 2 masses/2(dth_gen), 3 masses/2(dth_gen), 4 masses/2(dth_gen)
  1 mass/3(Tm_gen) -> Multiport Switch2/2
  ctrl4/1 -> Multiport Switch1/1, Multiport Switch2/1, Multiport Switch3/1
  2 masses/3(Tm_gen) -> Multiport Switch2/3
  3 masses/3(Tm_gen) -> Multiport Switch2/4
  4 masses/3(Tm_gen) -> Multiport Switch2/5
  ctrl2/1 -> 4 masses/Enable
  ctrl3/1 -> 3 masses/Enable
  1 mass/2(dw_5-2) -> Multiport Switch3/2
  2 masses/2(dw_5-2) -> Multiport Switch3/3
  ctrl7/1 -> 1 mass/Enable
  ctrl6/1 -> 2 masses/Enable
  3 masses/2(dw_5-2) -> Multiport Switch3/4
  Multiport Switch1/1 -> Tr2-5/1
  Multiport Switch2/1 -> Tm_g/1
  Multiport Switch3/1 -> dw_5-2/1
  4 masses/2(dw_5-2) -> Multiport Switch3/5

== system powerlib2/Machines/STG/speed regulator ==
  flowHP : Inport  Port=1  LatchInput=off
  Pref : Inport  Port=2  LatchInput=off
  wref : Inport  Port=3  LatchInput=off
  w : Inport  Port=4  LatchInput=off
  Dead Zone : DeadZone  LowerValue=-Dz  UpperValue=Dz  SaturateOnIntegerOverflow=on
  Gain : Gain  Gain=1/Rp  SaturateOnIntegerOverflow=on
  Gain1 : Gain  Gain=Kp  SaturateOnIntegerOverflow=on
  Gain2 : Gain  Orientation=up  Gain=Kp-1  SaturateOnIntegerOverflow=on
  Gain3 : Gain  Gain=1/Tsm  SaturateOnIntegerOverflow=on
  Gain4 : Gain  Gain=1/Rp  SaturateOnIntegerOverflow=on
  Servo-motor position : Integrator  InitialCondition=g0  LimitOutput=on  UpperSaturationLimit=gmax  LowerSaturationLimit=gmin
  Servo-motor speed limits : Saturate  UpperLimit=vgmax  LowerLimit=vgmin
  Speed Relay : simulink_extras/Additional Linear/Transfer Fcn (with initial outputs)  N=[1]  D=[Tsr 1]  Y0=g0  U0=g0
  Sum1 : Sum  Inputs=|+-  SaturateOnIntegerOverflow=on  InputSameDT=on
  Sum2 : Sum  Inputs=|+-  SaturateOnIntegerOverflow=on  InputSameDT=on
  Sum3 : Sum  Inputs=++-  SaturateOnIntegerOverflow=on  InputSameDT=on
  gate opening : Outport
  wires:
  Servo-motor speed limits/1 -> Servo-motor position/1
  Gain3/1 -> Servo-motor speed limits/1
  Sum2/1 -> Gain3/1
  Speed Relay/1 -> Sum2/1
  Sum1/1 -> Speed Relay/1
  Gain2/1 -> Sum1/2
  Gain1/1 -> Sum1/1
  Dead Zone/1 -> Gain1/1
  wref/1 -> Gain4/1
  Sum3/1 -> Dead Zone/1
  w/1 -> Gain/1
  Gain/1 -> Sum3/3
  Pref/1 -> Sum3/1
  Gain4/1 -> Sum3/2
  flowHP/1 -> Gain2/1
  Servo-motor position/1 -> gate opening/1, Sum2/2

== system powerlib2/Machines/STG/steam turbine ==
  gate : Inport  Port=1  LatchInput=off
  Pboil : Inport  Port=2  LatchInput=off
  Gain : Gain  Gain=F2  SaturateOnIntegerOverflow=on
  Gain2 : Gain  Gain=F3  SaturateOnIntegerOverflow=on
  Gain3 : Gain  Gain=F4  SaturateOnIntegerOverflow=on
  Gain4 : Gain  Gain=F5  SaturateOnIntegerOverflow=on
  Mux : Mux
  Product : Product  SaturateOnIntegerOverflow=on  InputSameDT=on
  Stage1 : Subsystem
  Stage2 : Subsystem
  "Stage3 " : Subsystem
  Stage4 : Subsystem
  flowHp : Outport
  T5-2 : Outport  Port=2
  wires:
  Mux/1 -> T5-2/1
  Stage4/1(Out1) -> Gain/1
  "Stage3 "/1(Out1) -> Stage4/1(In1), Gain2/1
  Gain/1 -> Mux/4
  Gain2/1 -> Mux/3
  Gain3/1 -> Mux/2
  Gain4/1 -> Mux/1
  Stage2/1(Out1) -> "Stage3 "/1(In1), Gain3/1
  Product/1 -> Stage1/1(In1)
  Stage1/1(Out1) -> flowHp/1, Stage2/1(In1), Gain4/1
  gate/1 -> Product/1
  Pboil/1 -> Product/2

== system powerlib2/Measurements/Multimeter/Phasor Measurements ==
  In1 : Inport  Port=1  LatchInput=off
  Enable : EnablePort
  180/pi : Gain  Gain=180/pi  SaturateOnIntegerOverflow=on
  Complex to Magnitude-Angle : ComplexToMagnitudeAngle
  Complex to Real-Imag : ComplexToRealImag
  Mux2 : Mux  Inputs=5
  Selector : Selector  Elements=OutputSelection  InputPortWidth=5*length(sel)
  Out1 : Outport  InitialOutput=0
  wires:
  In1/1 -> Mux2/1, Complex to Real-Imag/1, Complex to Magnitude-Angle/1
  Complex to Magnitude-Angle/2 -> 180/pi/1
  180/pi/1 -> Mux2/5
  Complex to Magnitude-Angle/1 -> Mux2/4
  Complex to Real-Imag/2 -> Mux2/3
  Complex to Real-Imag/1 -> Mux2/2
  Mux2/1 -> Selector/1
  Selector/1 -> Out1/1

== system powerlib2/Measurements/Multimeter/StoreData ==
  In1 : Inport  Port=1  LatchInput=off
  Enable : EnablePort
  To Workspace : ToWorkspace  VariableName=tp200592  SampleTime=-1  SaveFormat=Structure With Time
      settings: InitFcn=tag=strrep(tempname,tempdir,'');set_param(gcb,'VariableName',tag);clear tag;
  wires:
  In1/1 -> To Workspace/1

== system powerlib2/Measurements/Three-Phase V-I Measurement/Ia ==
  Out1 : Outport
  wires:
  [fkjhwerui] -> Out1/1

== system powerlib2/Measurements/Three-Phase V-I Measurement/Ib ==
  Out1 : Outport
  wires:
  [jhnfgjohfg] -> Out1/1

== system powerlib2/Measurements/Three-Phase V-I Measurement/Ic ==
  Out1 : Outport
  wires:
  [dsuiohew] -> Out1/1

== system powerlib2/Measurements/Three-Phase V-I Measurement/Phasor Measurements ==
  In1 : Inport  Port=1  LatchInput=off
  Enable : EnablePort
  180/pi : Gain  Gain=180/pi  SaturateOnIntegerOverflow=on
  Complex to Magnitude-Angle : ComplexToMagnitudeAngle
  Complex to Real-Imag : ComplexToRealImag
  Mux2 : Mux  Inputs=5
  Selector : Selector  Elements=OutputSelection  InputPortWidth=30
  Out1 : Outport  InitialOutput=0
  wires:
  Selector/1 -> Out1/1
  Mux2/1 -> Selector/1
  Complex to Real-Imag/1 -> Mux2/2
  Complex to Real-Imag/2 -> Mux2/3
  Complex to Magnitude-Angle/1 -> Mux2/4
  180/pi/1 -> Mux2/5
  Complex to Magnitude-Angle/2 -> 180/pi/1
  In1/1 -> Complex to Magnitude-Angle/1, Complex to Real-Imag/1, Mux2/1

== system powerlib2/Measurements/Three-Phase V-I Measurement/Vb ==
  Out1 : Outport
  wires:
  [gfgfger] -> Out1/1

== system powerlib2/Measurements/Three-Phase V-I Measurement/Vc ==
  Out1 : Outport
  wires:
  [tp1234] -> Out1/1

== system powerlib2/Measurements/Voltage Measurement/Phasor Measurements ==
  measure : Inport  Port=1  LatchInput=off
  Enable : EnablePort
  180/pi : Gain  Gain=180/pi  SaturateOnIntegerOverflow=on
  Complex to Magnitude-Angle : ComplexToMagnitudeAngle
  Complex to Real-Imag : ComplexToRealImag
  Mux2 : Mux  Inputs=5
  Selector : Selector  Elements=OutputSelection  InputPortWidth=5
  options : Outport  InitialOutput=0
  wires:
  Mux2/1 -> Selector/1
  measure/1 -> Complex to Magnitude-Angle/1, Complex to Real-Imag/1, Mux2/1
  Complex to Real-Imag/1 -> Mux2/2
  Complex to Real-Imag/2 -> Mux2/3
  Complex to Magnitude-Angle/1 -> Mux2/4
  Complex to Magnitude-Angle/2 -> 180/pi/1
  180/pi/1 -> Mux2/5
  Selector/1 -> options/1

== system powerlib2/Electrical Sources/3-Phase  Programmable  Voltage Source/Source/Harmonic A generation ==
  Enable : Inport  Port=1  LatchInput=off
  Gain2 : Gain  Gain=2*pi*n_Harmo  SaturateOnIntegerOverflow=on
  Gain3 : Gain  Gain=pi/180  SaturateOnIntegerOverflow=on
  Multiport Switch : MultiPortSwitch  Inputs=3  InputSameDT=on
  Negative-sequence : Constant  Value=[0 2*pi/3 -2*pi/3]
  Phase_Harmo : Constant  Value=Phase_Harmo
  Phase_Harmo1 : Constant  Value=Mag_Harmo
  Phase_Harmo2 : Constant  Value=Seq_Harmo
  Positive-sequence : Constant  Value=[0 -2*pi/3 2*pi/3]
  Product : Product  SaturateOnIntegerOverflow=on  InputSameDT=on
  Product1 : Product  Inputs=3  SaturateOnIntegerOverflow=on  InputSameDT=on
  Sum : Sum  Inputs=+++  SaturateOnIntegerOverflow=on  InputSameDT=on
  Sum1 : Sum  SaturateOnIntegerOverflow=on  InputSameDT=on
  Trigonometric Function1 : Trigonometry
  Zero-sequence : Constant  Value=[0 0 0]
  t : DigitalClock  SampleTime=Ts
  valp_nom1 : Constant  Value=Freq_Vps
  valp_nom2 : Constant
  HarmoA : Outport
  wires:
  Sum/1 -> Trigonometric Function1/1
  Multiport Switch/1 -> Sum/3
  Zero-sequence/1 -> Multiport Switch/2
  Positive-sequence/1 -> Multiport Switch/3
  Negative-sequence/1 -> Multiport Switch/4
  valp_nom1/1 -> Gain2/1
  Gain2/1 -> Product/2
  t/1 -> Product/1
  Product/1 -> Sum/1
  Trigonometric Function1/1 -> Product1/3
  Product1/1 -> HarmoA/1
  Phase_Harmo1/1 -> Product1/2
  Sum1/1 -> Multiport Switch/1
  Phase_Harmo2/1 -> Sum1/1
  valp_nom2/1 -> Sum1/2
  Enable/1 -> Product1/1
  Phase_Harmo/1 -> Gain3/1
  Gain3/1 -> Sum/2

== system powerlib2/Electrical Sources/3-Phase  Programmable  Voltage Source/Source/Harmonic B generation ==
  Enable : Inport  Port=1  LatchInput=off
  Gain2 : Gain  Gain=2*pi*n_Harmo  SaturateOnIntegerOverflow=on
  Gain3 : Gain  Gain=pi/180  SaturateOnIntegerOverflow=on
  Multiport Switch : MultiPortSwitch  Inputs=3  InputSameDT=on
  Negative-sequence : Constant  Value=[0 2*pi/3 -2*pi/3]
  Phase_Harmo : Constant  Value=Phase_Harmo
  Phase_Harmo1 : Constant  Value=Mag_Harmo
  Phase_Harmo2 : Constant  Value=Seq_Harmo
  Positive-sequence : Constant  Value=[0 -2*pi/3 2*pi/3]
  Product : Product  SaturateOnIntegerOverflow=on  InputSameDT=on
  Product1 : Product  Inputs=3  SaturateOnIntegerOverflow=on  InputSameDT=on
  Sum : Sum  Inputs=+++  SaturateOnIntegerOverflow=on  InputSameDT=on
  Sum1 : Sum  SaturateOnIntegerOverflow=on  InputSameDT=on
  Trigonometric Function1 : Trigonometry
  Zero-sequence : Constant  Value=[0 0 0]
  t : DigitalClock  SampleTime=Ts
  valp_nom1 : Constant  Value=Freq_Vps
  valp_nom2 : Constant
  HarmoB : Outport
  wires:
  Enable/1 -> Product1/1
  valp_nom2/1 -> Sum1/2
  Phase_Harmo2/1 -> Sum1/1
  Sum1/1 -> Multiport Switch/1
  Phase_Harmo1/1 -> Product1/2
  Product1/1 -> HarmoB/1
  Trigonometric Function1/1 -> Product1/3
  Product/1 -> Sum/1
  t/1 -> Product/1
  Gain2/1 -> Product/2
  valp_nom1/1 -> Gain2/1
  Negative-sequence/1 -> Multiport Switch/4
  Positive-sequence/1 -> Multiport Switch/3
  Zero-sequence/1 -> Multiport Switch/2
  Multiport Switch/1 -> Sum/3
  Sum/1 -> Trigonometric Function1/1
  Phase_Harmo/1 -> Gain3/1
  Gain3/1 -> Sum/2

== system powerlib2/Electrical Sources/3-Phase  Programmable  Voltage Source/Source/Timer ==
  Clock : Clock
  Look-Up Table : Lookup  DialogController=Simulink.DDGSource  InputValues=tv  OutputValues=opv  SaturateOnIntegerOverflow=on
  Out : Outport
  wires:
  Clock/1 -> Look-Up Table/1
  Look-Up Table/1 -> Out/1

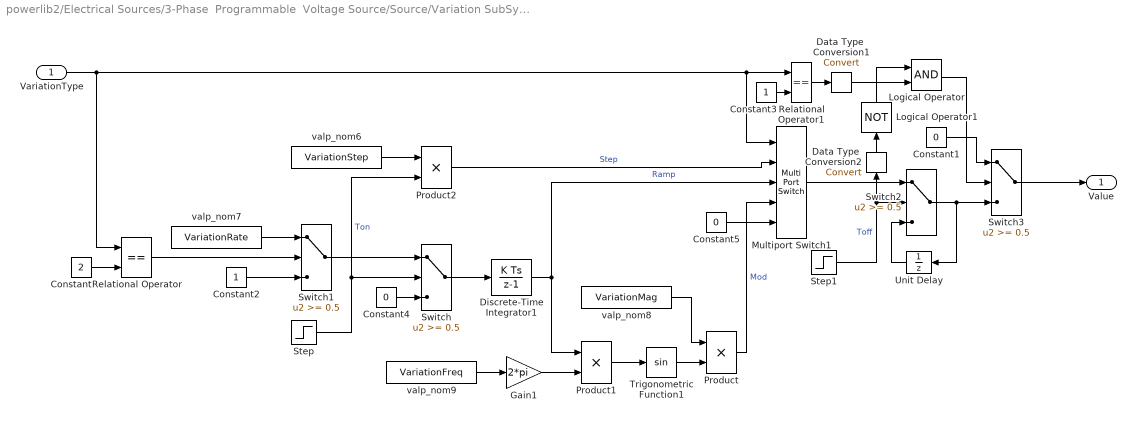
== system powerlib2/Electrical Sources/3-Phase  Programmable  Voltage Source/Source/Variation SubSystem ==
  VariationType : Inport  Port=1  LatchInput=off
  Constant : Constant  Value=2
  Constant1 : Constant  Value=0
  Constant2 : Constant
  Constant3 : Constant
  Constant4 : Constant  Value=0
  Constant5 : Constant  Value=0
  Data Type  Conversion1 : DataTypeConversion  OutDataTypeMode=boolean  SaturateOnIntegerOverflow=on  RndMeth=Zero
  Data Type  Conversion2 : DataTypeConversion  Orientation=up  OutDataTypeMode=boolean  SaturateOnIntegerOverflow=on  RndMeth=Zero
  Discrete-Time Integrator1 : DiscreteIntegrator  SampleTime=Ts  ICPrevOutput=DiscIntNeverNeededParam  ICPrevScaledInput=DiscIntNeverNeededParam
  Gain1 : Gain  Gain=2*pi  SaturateOnIntegerOverflow=on
  Logical Operator : Logic
  Logical Operator1 : Logic  Orientation=up  Operator=NOT
  Multiport Switch1 : MultiPortSwitch  InputSameDT=on
  Product : Product  SaturateOnIntegerOverflow=on  InputSameDT=on
  Product1 : Product  SaturateOnIntegerOverflow=on  InputSameDT=on
  Product2 : Product  SaturateOnIntegerOverflow=on  InputSameDT=on
  Relational Operator : RelationalOperator  Operator===  InputSameDT=on
  Relational Operator1 : RelationalOperator  Operator===  InputSameDT=on
  Step : Step  Time=Ton_Variation  SampleTime=Ts
  Step1 : Step  Time=Toff_Variation  Before=1  After=0  SampleTime=Ts
  Switch{,1..3} (4 alike) : Switch  Threshold=0.5  InputSameDT=on
  Trigonometric Function1 : Trigonometry
  Unit Delay : UnitDelay  Orientation=left  SampleTime=Ts
  valp_nom6 : Constant  Value=VariationStep
  valp_nom7 : Constant  Value=VariationRate
  valp_nom8 : Constant  Value=VariationMag
  valp_nom9 : Constant  Value=VariationFreq
  Value : Outport
  wires:
  Relational Operator1/1 -> Data Type  Conversion1/1
  Data Type  Conversion2/1 -> Logical Operator1/1
  Trigonometric Function1/1 -> Product/2
  valp_nom8/1 -> Product/1
  valp_nom9/1 -> Gain1/1
  Gain1/1 -> Product1/2
  Product1/1 -> Trigonometric Function1/1
  Product/1 -> Multiport Switch1/4  "Mod"
  valp_nom7/1 -> Switch1/1
  Constant2/1 -> Switch1/3
  Constant4/1 -> Switch/3
  Switch1/1 -> Switch/1
  Constant/1 -> Relational Operator/2
  Switch/1 -> Discrete-Time Integrator1/1
  Relational Operator/1 -> Switch1/2
  valp_nom6/1 -> Product2/1
  Product2/1 -> Multiport Switch1/2  "Step"
  Discrete-Time Integrator1/1 -> Product1/1, Multiport Switch1/3  "Ramp"
  VariationType/1 -> Multiport Switch1/1, Relational Operator1/1, Relational Operator/1
  Step/1 -> Switch/2, Product2/2  "Ton"
  Multiport Switch1/1 -> Switch2/1
  Unit Delay/1 -> Switch2/3
  Constant1/1 -> Switch3/1
  Switch2/1 -> Unit Delay/1, Switch3/3
  Switch3/1 -> Value/1
  Constant3/1 -> Relational Operator1/2
  Step1/1 -> Data Type  Conversion2/1, Switch2/2  "Toff"
  Logical Operator/1 -> Switch3/2
  Logical Operator1/1 -> Logical Operator/1
  Constant5/1 -> Multiport Switch1/5
  Data Type  Conversion1/1 -> Logical Operator/2

== system powerlib2/Machines/STG/4 mass shaft/1 mass ==
  Tt_1-4 : Inport  Port=1  LatchInput=off
  dth_gen : Inport  Port=2  LatchInput=off
  Enable : EnablePort
  Ground : Ground
  Ground1 : Ground  Orientation=left
  Mass2 : Subsystem  mask(Generic rotating mass){H=Ha(1), K=Ka(1), D=Da(1), dth0=dtha(1)}
      mask prompts: H "Inertia H (p.u.)"; K "Rigidity K (p.u.):"; D "Damping D (p.u.):"; dth0 "Initial angle deviation delta_theta (rad):"
  Mux : Mux  Inputs=[3 1]
  Mux1 : Mux  Inputs=[3 1]
  Selector : Selector  Elements=sel{1}  InputPortWidth=4
  Terminator : Terminator
  Ts_5-2 : Outport
  dw_5-2 : Outport  Port=2  InitialOutput=[0 0 0 0]
  Tm_gen : Outport  Port=3
  wires:
  Mass2/2(Ts_k) -> Tm_gen/1, Mux/2
  dth_gen/1 -> Mass2/3(deltat_k-1)
  Mass2/1(deltat_k) -> Terminator/1
  Ground/1 -> Mass2/1(Ts_k+1)
  Selector/1 -> Mass2/2(Tt_k)
  Mux/1 -> Ts_5-2/1
  Tt_1-4/1 -> Selector/1
  Ground1/1 -> Mux/1, Mux1/1
  Mass2/3(dw) -> Mux1/2
  Mux1/1 -> dw_5-2/1

== system powerlib2/Machines/STG/4 mass shaft/2 masses ==
  Tt_1-4 : Inport  Port=1  LatchInput=off
  dth_gen : Inport  Port=2  LatchInput=off
  Enable : EnablePort
  Demux : Demux  Outputs=2
  Ground : Ground
  Ground1 : Ground  Orientation=left
  Mass2 : Subsystem  mask(Generic rotating mass){H=Ha(1), K=Ka(1), D=Da(1), dth0=dtha(1)}
      mask prompts: H "Inertia H (p.u.)"; K "Rigidity K (p.u.):"; D "Damping D (p.u.):"; dth0 "Initial angle deviation delta_theta (rad):"
  Mass3 : Subsystem  mask(Generic rotating mass){H=Ha(2), K=Ka(2), D=Da(2), dth0=dtha(2)}
      mask prompts: H "Inertia H (p.u.)"; K "Rigidity K (p.u.):"; D "Damping D (p.u.):"; dth0 "Initial angle deviation delta_theta (rad):"
  Mux : Mux  Inputs=[ 2 1 1 ]
  Mux1 : Mux  Inputs=[ 2 1 1 ]
  Selector : Selector  Elements=sel{2}  InputPortWidth=4
  Terminator : Terminator
  Ts_5-2 : Outport
  dw_5-2 : Outport  Port=2  InitialOutput=[0 0 0 0]
  Tm_gen : Outport  Port=3
  wires:
  Mass2/2(Ts_k) -> Tm_gen/1, Mux/3
  dth_gen/1 -> Mass2/3(deltat_k-1)
  Mass2/1(deltat_k) -> Mass3/3(deltat_k-1)
  Demux/2 -> Mass2/2(Tt_k)
  Ground/1 -> Mass3/1(Ts_k+1)
  Mass3/1(deltat_k) -> Terminator/1
  Mass3/2(Ts_k) -> Mass2/1(Ts_k+1), Mux/2
  Mux/1 -> Ts_5-2/1
  Selector/1 -> Demux/1
  Tt_1-4/1 -> Selector/1
  Demux/1 -> Mass3/2(Tt_k)
  Ground1/1 -> Mux/1, Mux1/1
  Mux1/1 -> dw_5-2/1
  Mass3/3(dw) -> Mux1/2
  Mass2/3(dw) -> Mux1/3

== system powerlib2/Machines/STG/4 mass shaft/3 masses ==
  Tt_1-4 : Inport  Port=1  LatchInput=off
  dth_gen : Inport  Port=2  LatchInput=off
  Enable : EnablePort
  Demux : Demux  Outputs=3
  Ground : Ground
  Ground1 : Ground  Orientation=left
  Mass2 : Subsystem  mask(Generic rotating mass){H=Ha(1), K=Ka(1), D=Da(1), dth0=dtha(1)}
      mask prompts: H "Inertia H (p.u.)"; K "Rigidity K (p.u.):"; D "Damping D (p.u.):"; dth0 "Initial angle deviation delta_theta (rad):"
  Mass3 : Subsystem  mask(Generic rotating mass){H=Ha(2), K=Ka(2), D=Da(2), dth0=dtha(2)}
      mask prompts: H "Inertia H (p.u.)"; K "Rigidity K (p.u.):"; D "Damping D (p.u.):"; dth0 "Initial angle deviation delta_theta (rad):"
  Mass4 : Subsystem  mask(Generic rotating mass){H=Ha(3), K=Ka(3), D=Da(3), dth0=dtha(3)}
      mask prompts: H "Inertia H (p.u.)"; K "Rigidity K (p.u.):"; D "Damping D (p.u.):"; dth0 "Initial angle deviation delta_theta (rad):"
  Mux : Mux
  Mux1 : Mux
  Selector : Selector  Elements=sel{3}  InputPortWidth=4
  Terminator : Terminator
  Ts_5-2 : Outport
  dw_5-2 : Outport  Port=2  InitialOutput=[0 0 0 0]
  Tm_gen : Outport  Port=3
  wires:
  Mass3/2(Ts_k) -> Mass2/1(Ts_k+1), Mux/3
  Tt_1-4/1 -> Selector/1
  Selector/1 -> Demux/1
  Mass2/2(Ts_k) -> Mux/4, Tm_gen/1
  dth_gen/1 -> Mass2/3(deltat_k-1)
  Mass4/1(deltat_k) -> Terminator/1
  Ground/1 -> Mass4/1(Ts_k+1)
  Demux/1 -> Mass4/2(Tt_k)
  Demux/2 -> Mass3/2(Tt_k)
  Demux/3 -> Mass2/2(Tt_k)
  Mass2/1(deltat_k) -> Mass3/3(deltat_k-1)
  Mass3/1(deltat_k) -> Mass4/3(deltat_k-1)
  Mass4/2(Ts_k) -> Mass3/1(Ts_k+1), Mux/2
  Mass4/3(dw) -> Mux1/2
  Mass3/3(dw) -> Mux1/3
  Mux/1 -> Ts_5-2/1
  Ground1/1 -> Mux/1, Mux1/1
  Mux1/1 -> dw_5-2/1
  Mass2/3(dw) -> Mux1/4

== system powerlib2/Machines/STG/4 mass shaft/4 masses ==
  Tt_1-4 : Inport  Port=1  LatchInput=off
  dth_gen : Inport  Port=2  LatchInput=off
  Enable : EnablePort
  Demux : Demux
  Ground : Ground
  Mass2 : Subsystem  mask(Generic rotating mass){H=Ha(1), K=Ka(1), D=Da(1), dth0=dtha(1)}
      mask prompts: H "Inertia H (p.u.)"; K "Rigidity K (p.u.):"; D "Damping D (p.u.):"; dth0 "Initial angle deviation delta_theta (rad):"
  Mass3 : Subsystem  mask(Generic rotating mass){H=Ha(2), K=Ka(2), D=Da(2), dth0=dtha(2)}
      mask prompts: H "Inertia H (p.u.)"; K "Rigidity K (p.u.):"; D "Damping D (p.u.):"; dth0 "Initial angle deviation delta_theta (rad):"
  Mass4 : Subsystem  mask(Generic rotating mass){H=Ha(3), K=Ka(3), D=Da(3), dth0=dtha(3)}
      mask prompts: H "Inertia H (p.u.)"; K "Rigidity K (p.u.):"; D "Damping D (p.u.):"; dth0 "Initial angle deviation delta_theta (rad):"
  Mass5 : Subsystem  mask(Generic rotating mass){H=Ha(4), K=Ka(4), D=Da(4), dth0=dtha(4)}
      mask prompts: H "Inertia H (p.u.)"; K "Rigidity K (p.u.):"; D "Damping D (p.u.):"; dth0 "Initial angle deviation delta_theta (rad):"
  Mux : Mux
  Mux1 : Mux
  Terminator : Terminator
  Ts_5-2 : Outport
  dw_5-2 : Outport  Port=2  InitialOutput=[0 0 0 0]
  Tm_gen : Outport  Port=3
  wires:
  Mass2/2(Ts_k) -> Tm_gen/1, Mux/4
  dth_gen/1 -> Mass2/3(deltat_k-1)
  Tt_1-4/1 -> Demux/1
  Mass3/2(Ts_k) -> Mux/3, Mass2/1(Ts_k+1)
  Mass4/2(Ts_k) -> Mux/2, Mass3/1(Ts_k+1)
  Mass5/2(Ts_k) -> Mass4/1(Ts_k+1), Mux/1
  Mass4/1(deltat_k) -> Mass5/3(deltat_k-1)
  Mass3/1(deltat_k) -> Mass4/3(deltat_k-1)
  Mass2/1(deltat_k) -> Mass3/3(deltat_k-1)
  Demux/4 -> Mass2/2(Tt_k)
  Demux/3 -> Mass3/2(Tt_k)
  Demux/2 -> Mass4/2(Tt_k)
  Demux/1 -> Mass5/2(Tt_k)
  Ground/1 -> Mass5/1(Ts_k+1)
  Mass5/1(deltat_k) -> Terminator/1
  Mux/1 -> Ts_5-2/1
  Mass5/3(dw) -> Mux1/1
  Mass4/3(dw) -> Mux1/2
  Mux1/1 -> dw_5-2/1
  Mass3/3(dw) -> Mux1/3
  Mass2/3(dw) -> Mux1/4

== system powerlib2/Machines/STG/steam turbine/Stage1 ==
  In1 : Inport  Port=1  LatchInput=off
  Constant1 : Constant  Orientation=down  Value=Ta(4)~=0
  Stage4 : Subsystem  TreatAsAtomicUnit=on
  Switch3 : Switch  Threshold=0.5  InputSameDT=on
  Out1 : Outport
  wires:
  Switch3/1 -> Out1/1
  In1/1 -> Switch3/3, Stage4/1(In1)
  Constant1/1 -> Switch3/2, Stage4/Enable
  Stage4/1(Out1) -> Switch3/1

== system powerlib2/Machines/STG/steam turbine/Stage2 ==
  In1 : Inport  Port=1  LatchInput=off
  Constant2 : Constant  Orientation=down  Value=Ta(3)~=0
  Stage3 : Subsystem  TreatAsAtomicUnit=on
  Switch2 : Switch  Threshold=0.5  InputSameDT=on
  Out1 : Outport
  wires:
  In1/1 -> Switch2/3, Stage3/1(In1)
  Switch2/1 -> Out1/1
  Constant2/1 -> Switch2/2, Stage3/Enable
  Stage3/1(Out1) -> Switch2/1

== system powerlib2/Machines/STG/steam turbine/Stage3  ==
  In1 : Inport  Port=1  LatchInput=off
  Constant3 : Constant  Orientation=down  Value=Ta(2)~=0
  Stage2 : Subsystem  TreatAsAtomicUnit=on
  Switch1 : Switch  Threshold=0.5  InputSameDT=on
  Out1 : Outport
  wires:
  In1/1 -> Switch1/3, Stage2/1(In1)
  Switch1/1 -> Out1/1
  Constant3/1 -> Switch1/2, Stage2/Enable
  Stage2/1(Out1) -> Switch1/1

== system powerlib2/Machines/STG/steam turbine/Stage4 ==
  In1 : Inport  Port=1  LatchInput=off
  Constant4 : Constant  Orientation=down  Value=Ta(1)~=0
  Stage1 : Subsystem  TreatAsAtomicUnit=on
  Switch : Switch  Threshold=0.5  InputSameDT=on
  Out1 : Outport
  wires:
  Switch/1 -> Out1/1
  Stage1/1(Out1) -> Switch/1
  In1/1 -> Switch/3, Stage1/1(In1)
  Constant4/1 -> Switch/2, Stage1/Enable

== system powerlib2/Machines/STG/4 mass shaft/1 mass/Mass2 ==
  Ts_k+1 : Inport  Port=1  LatchInput=off
  Tt_k : Inport  Port=2  LatchInput=off
  deltat_k-1 : Inport  Port=3  LatchInput=off
  Gain10 : Gain  Gain=D  SaturateOnIntegerOverflow=on
  Gain11 : Gain  Gain=K  SaturateOnIntegerOverflow=on
  Gain9 : Gain  Gain=1/(2*H)  SaturateOnIntegerOverflow=on
  Integrator6 : Integrator
  Integrator7 : Integrator  InitialCondition=dth0
  Sum11 : Sum  Orientation=left  Inputs=|+-  SaturateOnIntegerOverflow=on  InputSameDT=on
  Sum9 : Sum  Inputs=+|+|-|-  SaturateOnIntegerOverflow=on  InputSameDT=on
  pu2radpersec : Gain  Gain=120*pi  SaturateOnIntegerOverflow=on
  deltat_k : Outport  InitialOutput=0
  Ts_k : Outport  Port=2  InitialOutput=0
  dw : Outport  Port=3  InitialOutput=0
  wires:
  deltat_k-1/1 -> Sum11/2
  Sum11/1 -> Gain11/1
  Integrator7/1 -> deltat_k/1, Sum11/1
  pu2radpersec/1 -> Integrator7/1
  Integrator6/1 -> pu2radpersec/1, Gain10/1, dw/1
  Tt_k/1 -> Sum9/2
  Sum9/1 -> Gain9/1
  Gain10/1 -> Sum9/4
  Gain11/1 -> Ts_k/1, Sum9/3
  Ts_k+1/1 -> Sum9/1
  Gain9/1 -> Integrator6/1
